simulink library "csu_cfe_cfe_time_lib"  (R2014b)
settings: Solver=ode45  StartTime=0.0  StopTime=10.0  RelTol=1e-3
undefined symbols (not defined in the file or in its folder): cfe_initial_utc_time
undefined symbols (not defined in the file): fsw_dt
libraries: util_info_lib x1
settings Model: Creator=mstewart  LastModifiedBy=mstewart

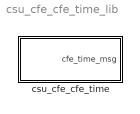
== system csu_cfe_cfe_time_lib ==
  csu_cfe_cfe_time : Subsystem  mask{sch_dt=fsw_dt}
      mask prompts: sch_dt "Sample Time"

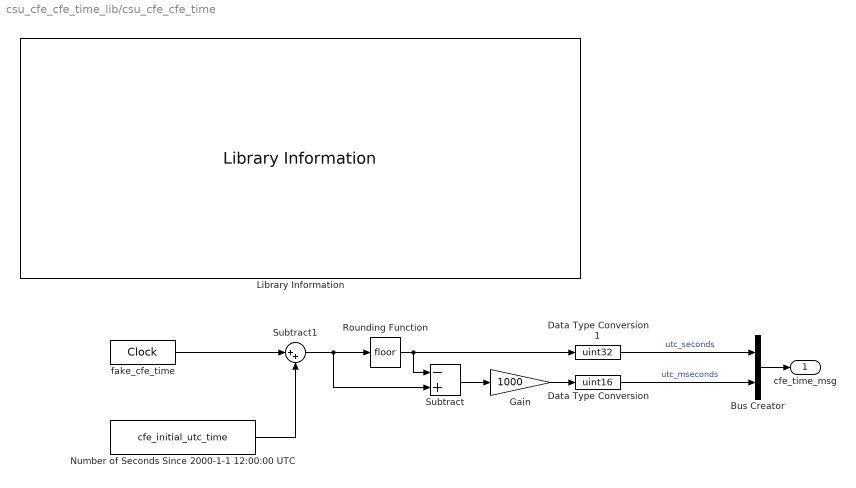
== system csu_cfe_cfe_time_lib/csu_cfe_cfe_time ==
  Bus Creator : BusCreator  Inputs=2  OutDataTypeStr=Bus: cfe_time_msg  NonVirtualBus=on
  Data Type Conversion : DataTypeConversion  OutDataTypeStr=uint16  RndMeth=Round
  Data Type Conversion1 : DataTypeConversion  OutDataTypeStr=uint32
  Gain : Gain  Gain=1000
  Library Information : util_info_lib/Library Information  owner='NONE'
  Number of Seconds Since 2000-1-1 12:00:00 UTC : Constant  Description=|  Value=cfe_initial_utc_time
      | Number of Seconds                   
      | July 4, 2014 22:40:00 UTC           
      | Calculate on Web Site:              
      | www.mbari.org/staff/rich/utccalc.htm
  Rounding Function : Rounding
  Subtract : Sum  Inputs=-+
  Subtract1 : Sum  Inputs=|++
  fake_cfe_time : DigitalClock  SampleTime=sch_dt
  cfe_time_msg : Outport  OutDataTypeStr=Bus: cfe_time_msg
  wires:
  Gain/1 -> Data Type Conversion/1
  Rounding Function/1 -> Data Type Conversion1/1, Subtract/1
  Subtract/1 -> Gain/1
  Bus Creator/1 -> cfe_time_msg/1
  Data Type Conversion/1 -> Bus Creator/2  "utc_mseconds"
  Data Type Conversion1/1 -> Bus Creator/1  "utc_seconds"
  fake_cfe_time/1 -> Subtract1/1
  Number of Seconds Since 2000-1-1 12:00:00 UTC/1 -> Subtract1/2
  Subtract1/1 -> Subtract/2, Rounding Function/1
